simulink model "Plant_Model"  (R2022b)
settings: Solver=VariableStepAuto  StartTime=0.0  StopTime=1000  RelTol=1e-3
settings Model: Creator=Fatha  LastModifiedBy=yonat
settings DebuggingCC: UnconnectedInputMsg=warning  UnconnectedOutputMsg=warning  UnconnectedLineMsg=warning
settings ModelReferenceCC: EnableRefExpFcnMdlSchedulingChecks=on
settings RTWCC: DLArmComputeVersion=19.05

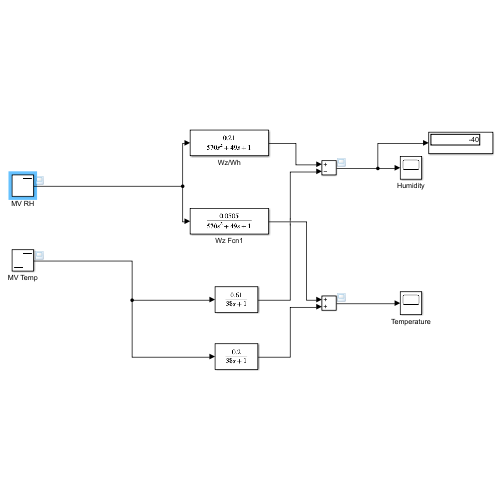
[thumbnail: Simulink's stored preview of the top-level diagram]
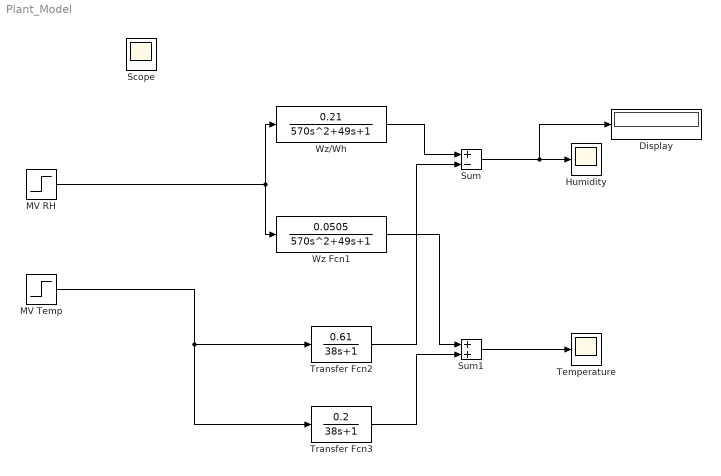
== system Plant_Model ==
  Display : Display
  Humidity : Scope
  MV RH : Step  Time=500  After=100  SampleTime=0
  MV Temp : Step  Time=500  After=100  SampleTime=0
  Sum : Sum  Inputs=+-
  Sum1 : Sum
  Temperature : Scope
  Transfer Fcn2 : TransferFcn  Numerator=[0.61]  Denominator=[38 1]
  Transfer Fcn3 : TransferFcn  Numerator=[0.2]  Denominator=[38 1]
  Wz Fcn1 : TransferFcn  Numerator=[0.0505]  Denominator=[570 49 1]
  Wz/Wh : TransferFcn  Numerator=[0.21]  Denominator=[570 49 1]
  Scope : Scope
  wires:
  Wz/Wh/1 -> Sum/1
  Transfer Fcn2/1 -> Sum/2
  Wz Fcn1/1 -> Sum1/1
  Transfer Fcn3/1 -> Sum1/2
  Sum1/1 -> Temperature/1
  Sum/1 -> Display/1, Humidity/1
  MV RH/1 -> Wz/Wh/1, Wz Fcn1/1
  MV Temp/1 -> Transfer Fcn3/1, Transfer Fcn2/1
